simulink library "inp"  (R2021b)
settings: Solver=VariableStepAuto  StartTime=0.0  StopTime=10.0  RelTol=1e-3
undefined symbols (not defined in the file): C_TASK_5MS_S, FALSE, KINP_AcoreReadyToSlp_flg_ovrdflg, KINP_AcoreReadyToSlp_flg_ovrdval, KINP_AllowMovThd_OTA_enum_ovrdflg, KINP_AllowMovThd_OTA_enum_ovrdval, KINP_APSAngleTarget_Deg_ovrdflg, KINP_APSAngleTarget_Deg_ovrdval, KINP_APSDecReq_mps2_ovrdflg, KINP_APSDecReq_mps2_ovrdval, KINP_APSDecReqA_flg_ovrdflg, KINP_APSDecReqA_flg_ovrdval, KINP_APSDFLL_cm_ovrdflg, KINP_APSDFLL_cm_ovrdval, KINP_APSDFLR_cm_ovrdflg, KINP_APSDFLR_cm_ovrdval, KINP_APSDRLL_cm_ovrdflg, KINP_APSDRLL_cm_ovrdval, KINP_APSDRLR_cm_ovrdflg, KINP_APSDRLR_cm_ovrdval, KINP_APSExitCondition_enum_ovrdflg, KINP_APSExitCondition_enum_ovrdval, KINP_APSHWVer_enum_ovrdflg, KINP_APSHWVer_enum_ovrdval, KINP_APSProgressPCT_pct_ovrdflg, KINP_APSProgressPCT_pct_ovrdval, KINP_APSPwrReq_enum_ovrdflg, KINP_APSPwrReq_enum_ovrdval, KINP_APSReq_enum_ovrdflg, KINP_APSReq_enum_ovrdval, KINP_APSRQDisplay_enum_ovrdflg, KINP_APSRQDisplay_enum_ovrdval, KINP_APSRqEPASCtrl_flg_ovrdflg, KINP_APSRqEPASCtrl_flg_ovrdval, KINP_APSShiftPosnReq_enum_ovrdval, KINP_APSShiftPosnReq_enum_ovrflg, KINP_APSSpeedCMD_kph_ovrdval, KINP_APSSpeedCMD_kph_ovrflg, KINP_APSStaSystem_enum_ovrdflg, KINP_APSStaSystem_enum_ovrdval, KINP_APSSWVer_enum_ovrdflg, KINP_APSSWVer_enum_ovrdval, KINP_APSVMCReqA_flg_ovrdval, KINP_APSVMCReqA_flg_ovrflg, KINP_APSVRqEPASCtrl_flg_ovrdflg, KINP_APSVRqEPASCtrl_flg_ovrdval, KINP_AuxBattVolmV_mV_ovrdflg, KINP_AuxBattVolmV_mV_ovrdval, KINP_CAASSta_enum_ovrdflg, KINP_CAASSta_enum_ovrdval, KINP_CAASVMCReqA_flg_ovrdval, KINP_CAASVMCReqA_flg_ovrflg, KINP_CAN1BusOff_flg_ovrdflg, KINP_CAN1BusOff_flg_ovrdval, KINP_CAN2BusOff_flg_ovrdflg, KINP_CAN2BusOff_flg_ovrdval, KINP_CAN3BusOff_flg_ovrdflg, KINP_CAN3BusOff_flg_ovrdval, KINP_CAN4BusOff_flg_ovrdflg, KINP_CAN4BusOff_flg_ovrdval ... (+152)
libraries: FVT_lib x1037, hcu_lib x1
(part 16 of 34)

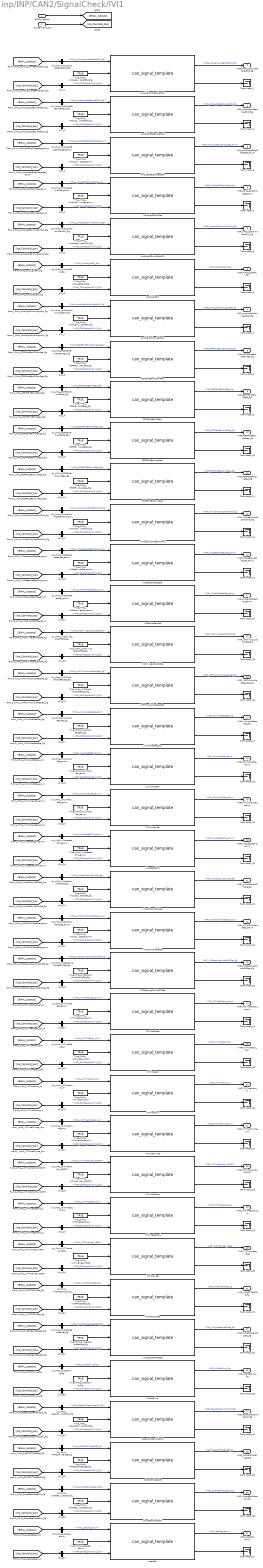
== system inp/INP/CAN2/SignalCheck/IVI1 ==
  BHAL_outputs : Inport
  inp_CanValid_bus : Inport  Port=2
  AmbLighLowBatAlertSW : FVT_lib/inp/can_signal_template  SystemSampleTime=-1  VariantActivationTime=update diagram  Latency=0  AutoFrameSizeCalculation=off
      link override defval: Value=KINP_AmbLighLowBatAlertSW_flg_defval
      link override ovrdflg: Value=KINP_AmbLighLowBatAlertSW_flg_ovrdflg
      link override ovrdval: Value=KINP_AmbLighLowBatAlertSW_flg_ovrdval
  AmbLighSafetyAlertSW : FVT_lib/inp/can_signal_template  SystemSampleTime=-1  VariantActivationTime=update diagram  Latency=0  AutoFrameSizeCalculation=off
      link override defval: Value=KINP_AmbLighSafetyAlertSW_flg_defval
      link override ovrdflg: Value=KINP_AmbLighSafetyAlertSW_flg_ovrdflg
      link override ovrdval: Value=KINP_AmbLighSafetyAlertSW_flg_ovrdval
  AmbLightBrightnessSet : FVT_lib/inp/can_signal_template  SystemSampleTime=-1  VariantActivationTime=update diagram  Latency=0  AutoFrameSizeCalculation=off
      link override defval: Value=KINP_AmbLightBrightnessSet_enum_defval
      link override ovrdflg: Value=KINP_AmbLightBrightnessSet_enum_ovrdflg
      link override ovrdval: Value=KINP_AmbLightBrightnessSet_enum_ovrdval
  AmbLightColorSet : FVT_lib/inp/can_signal_template  SystemSampleTime=-1  VariantActivationTime=update diagram  Latency=0  AutoFrameSizeCalculation=off
      link override defval: Value=KINP_AmbLightColorSet_enum_defval
      link override ovrdflg: Value=KINP_AmbLightColorSet_enum_ovrdflg
      link override ovrdval: Value=KINP_AmbLightColorSet_enum_ovrdval
  AmbLightDimInDarkSW : FVT_lib/inp/can_signal_template  SystemSampleTime=-1  VariantActivationTime=update diagram  Latency=0  AutoFrameSizeCalculation=off
      link override defval: Value=KINP_AmbLightDimInDarkSW_flg_defval
      link override ovrdflg: Value=KINP_AmbLightDimInDarkSW_flg_ovrdflg
      link override ovrdval: Value=KINP_AmbLightDimInDarkSW_flg_ovrdval
  AmbLightSW : FVT_lib/inp/can_signal_template  SystemSampleTime=-1  VariantActivationTime=update diagram  Latency=0  AutoFrameSizeCalculation=off
      link override defval: Value=KINP_AmbLightSW_flg_defval
      link override ovrdflg: Value=KINP_AmbLightSW_flg_ovrdflg
      link override ovrdval: Value=KINP_AmbLightSW_flg_ovrdval
  AmbLightWlcmLightSW : FVT_lib/inp/can_signal_template  SystemSampleTime=-1  VariantActivationTime=update diagram  Latency=0  AutoFrameSizeCalculation=off
      link override defval: Value=KINP_AmbLightWlcmLightSW_flg_defval
      link override ovrdflg: Value=KINP_AmbLightWlcmLightSW_flg_ovrdflg
      link override ovrdval: Value=KINP_AmbLightWlcmLightSW_flg_ovrdval
  FCPFrEvtBtnACMaxReq : FVT_lib/inp/can_signal_template  SystemSampleTime=-1  VariantActivationTime=update diagram  Latency=0  AutoFrameSizeCalculation=off
      link override defval: Value=KINP_FCPFrEvtBtnACMaxReq_flg_defval
      link override ovrdflg: Value=KINP_FCPFrEvtBtnACMaxReq_flg_ovrdflg
      link override ovrdval: Value=KINP_FCPFrEvtBtnACMaxReq_flg_ovrdval
  FCPFrEvtBtnACReq : FVT_lib/inp/can_signal_template  SystemSampleTime=-1  VariantActivationTime=update diagram  Latency=0  AutoFrameSizeCalculation=off
      link override defval: Value=KINP_FCPFrEvtBtnACReq_flg_defval
      link override ovrdflg: Value=KINP_FCPFrEvtBtnACReq_flg_ovrdflg
      link override ovrdval: Value=KINP_FCPFrEvtBtnACReq_flg_ovrdval
  FCPFrEvtBtnAutoReq : FVT_lib/inp/can_signal_template  SystemSampleTime=-1  VariantActivationTime=update diagram  Latency=0  AutoFrameSizeCalculation=off
      link override defval: Value=KINP_FCPFrEvtBtnAutoReq_flg_defval
      link override ovrdflg: Value=KINP_FCPFrEvtBtnAutoReq_flg_ovrdflg
      link override ovrdval: Value=KINP_FCPFrEvtBtnAutoReq_flg_ovrdval
  FCPFrEvtBtnSyncReq : FVT_lib/inp/can_signal_template  SystemSampleTime=-1  VariantActivationTime=update diagram  Latency=0  AutoFrameSizeCalculation=off
      link override defval: Value=KINP_FCPFrEvtBtnSyncReq_flg_defval
      link override ovrdflg: Value=KINP_FCPFrEvtBtnSyncReq_flg_ovrdflg
      link override ovrdval: Value=KINP_FCPFrEvtBtnSyncReq_flg_ovrdval
  IVIAutoWipHSpdSWCmd : FVT_lib/inp/can_signal_template  SystemSampleTime=-1  VariantActivationTime=update diagram  Latency=0  AutoFrameSizeCalculation=off
      link override defval: Value=KINP_IVIAutoWipHSpdSWCmd_flg_defval
      link override ovrdflg: Value=KINP_IVIAutoWipHSpdSWCmd_flg_ovrdflg
      link override ovrdval: Value=KINP_IVIAutoWipHSpdSWCmd_flg_ovrdval
  IVICreateAccReqSta : FVT_lib/inp/can_signal_template  SystemSampleTime=-1  VariantActivationTime=update diagram  Latency=0  AutoFrameSizeCalculation=off
      link override defval: Value=KINP_IVICreateAccReqSta_enum_defval
      link override ovrdflg: Value=KINP_IVICreateAccReqSta_enum_ovrdflg
      link override ovrdval: Value=KINP_IVICreateAccReqSta_enum_ovrdval
  IVIDelAccReqSta : FVT_lib/inp/can_signal_template  SystemSampleTime=-1  VariantActivationTime=update diagram  Latency=0  AutoFrameSizeCalculation=off
      link override defval: Value=KINP_IVIDelAccReqSta_enum_defval
      link override ovrdflg: Value=KINP_IVIDelAccReqSta_enum_ovrdflg
      link override ovrdval: Value=KINP_IVIDelAccReqSta_enum_ovrdval
  IVIDrivingLockSWSta : FVT_lib/inp/can_signal_template  SystemSampleTime=-1  VariantActivationTime=update diagram  Latency=0  AutoFrameSizeCalculation=off
      link override defval: Value=KINP_IVIDrivingLockSWSta_flg_defval
      link override ovrdflg: Value=KINP_IVIDrivingLockSWSta_flg_ovrdflg
      link override ovrdval: Value=KINP_IVIDrivingLockSWSta_flg_ovrdval
  IVIFrTrunkUnlockReqSta : FVT_lib/inp/can_signal_template  SystemSampleTime=-1  VariantActivationTime=update diagram  Latency=0  AutoFrameSizeCalculation=off
      link override defval: Value=KINP_IVIFrTrunkUnlockReqSta_flg_defval
      link override ovrdflg: Value=KINP_IVIFrTrunkUnlockReqSta_flg_ovrdflg
      link override ovrdval: Value=KINP_IVIFrTrunkUnlockReqSta_flg_ovrdval
  IVILinkAccReqSta : FVT_lib/inp/can_signal_template  SystemSampleTime=-1  VariantActivationTime=update diagram  Latency=0  AutoFrameSizeCalculation=off
      link override defval: Value=KINP_IVILinkAccReqSta_flg_defval
      link override ovrdflg: Value=KINP_IVILinkAccReqSta_flg_ovrdflg
      link override ovrdval: Value=KINP_IVILinkAccReqSta_flg_ovrdval
  IVILinkAccSta : FVT_lib/inp/can_signal_template  SystemSampleTime=-1  VariantActivationTime=update diagram  Latency=0  AutoFrameSizeCalculation=off
      link override defval: Value=KINP_IVILinkAccSta_enum_defval
      link override ovrdflg: Value=KINP_IVILinkAccSta_enum_ovrdflg
      link override ovrdval: Value=KINP_IVILinkAccSta_enum_ovrdval
  IVILinkKeySta : FVT_lib/inp/can_signal_template  SystemSampleTime=-1  VariantActivationTime=update diagram  Latency=0  AutoFrameSizeCalculation=off
      link override defval: Value=KINP_IVILinkKeySta_enum_defval
      link override ovrdflg: Value=KINP_IVILinkKeySta_enum_ovrdflg
      link override ovrdval: Value=KINP_IVILinkKeySta_enum_ovrdval
  IVILocatedSTA : FVT_lib/inp/can_signal_template  SystemSampleTime=-1  VariantActivationTime=update diagram  Latency=0  AutoFrameSizeCalculation=off
      link override defval: Value=KINP_IVILocatedSTA_enum_defval
      link override ovrdflg: Value=KINP_IVILocatedSTA_enum_ovrdflg
      link override ovrdval: Value=KINP_IVILocatedSTA_enum_ovrdval
  IVILockSoundSWSta : FVT_lib/inp/can_signal_template  SystemSampleTime=-1  VariantActivationTime=update diagram  Latency=0  AutoFrameSizeCalculation=off
      link override defval: Value=KINP_IVILockSoundSWSta_flg_defval
      link override ovrdflg: Value=KINP_IVILockSoundSWSta_flg_ovrdflg
      link override ovrdval: Value=KINP_IVILockSoundSWSta_flg_ovrdval
  IVISWCVibModeSta : FVT_lib/inp/can_signal_template  SystemSampleTime=-1  VariantActivationTime=update diagram  Latency=0  AutoFrameSizeCalculation=off
      link override defval: Value=KINP_IVISWCVibModeSta_enum_defval
      link override ovrdflg: Value=KINP_IVISWCVibModeSta_enum_ovrdflg
      link override ovrdval: Value=KINP_IVISWCVibModeSta_enum_ovrdval
  IVIStoppingUnlockSWSta : FVT_lib/inp/can_signal_template  SystemSampleTime=-1  VariantActivationTime=update diagram  Latency=0  AutoFrameSizeCalculation=off
      link override defval: Value=KINP_IVIStoppingUnlockSWSta_flg_defval
      link override ovrdflg: Value=KINP_IVIStoppingUnlockSWSta_flg_ovrdflg
      link override ovrdval: Value=KINP_IVIStoppingUnlockSWSta_flg_ovrdval
  IVITimeCheck : FVT_lib/inp/can_signal_template  SystemSampleTime=-1  VariantActivationTime=update diagram  Latency=0  AutoFrameSizeCalculation=off
      link override defval: Value=KINP_IVITimeCheck_enum_defval
      link override ovrdflg: Value=KINP_IVITimeCheck_enum_ovrdflg
      link override ovrdval: Value=KINP_IVITimeCheck_enum_ovrdval
  IVITimeDay : FVT_lib/inp/can_signal_template  SystemSampleTime=-1  VariantActivationTime=update diagram  Latency=0  AutoFrameSizeCalculation=off
      link override defval: Value=KINP_IVITimeDay_DAY_defval
      link override ovrdflg: Value=KINP_IVITimeDay_DAY_ovrdflg
      link override ovrdval: Value=KINP_IVITimeDay_DAY_ovrdval
  IVITimeHour : FVT_lib/inp/can_signal_template  SystemSampleTime=-1  VariantActivationTime=update diagram  Latency=0  AutoFrameSizeCalculation=off
      link override defval: Value=KINP_IVITimeHour_hr_defval
      link override ovrdflg: Value=KINP_IVITimeHour_hr_ovrdflg
      link override ovrdval: Value=KINP_IVITimeHour_hr_ovrdval
  IVITimeMinute : FVT_lib/inp/can_signal_template  SystemSampleTime=-1  VariantActivationTime=update diagram  Latency=0  AutoFrameSizeCalculation=off
      link override defval: Value=KINP_IVITimeMinute_min_defval
      link override ovrdflg: Value=KINP_IVITimeMinute_min_ovrdflg
      link override ovrdval: Value=KINP_IVITimeMinute_min_ovrdval
  IVITimeMonth : FVT_lib/inp/can_signal_template  SystemSampleTime=-1  VariantActivationTime=update diagram  Latency=0  AutoFrameSizeCalculation=off
      link override defval: Value=KINP_IVITimeMonth_MONTH_defval
      link override ovrdflg: Value=KINP_IVITimeMonth_MONTH_ovrdflg
      link override ovrdval: Value=KINP_IVITimeMonth_MONTH_ovrdval
  IVITimeSecond : FVT_lib/inp/can_signal_template  SystemSampleTime=-1  VariantActivationTime=update diagram  Latency=0  AutoFrameSizeCalculation=off
      link override defval: Value=KINP_IVITimeSecond_s_defval
      link override ovrdflg: Value=KINP_IVITimeSecond_s_ovrdflg
      link override ovrdval: Value=KINP_IVITimeSecond_s_ovrdval
  IVITimeYear : FVT_lib/inp/can_signal_template  SystemSampleTime=-1  VariantActivationTime=update diagram  Latency=0  AutoFrameSizeCalculation=off
      link override defval: Value=KINP_IVITimeYear_YEAR_defval
      link override ovrdflg: Value=KINP_IVITimeYear_YEAR_ovrdflg
      link override ovrdval: Value=KINP_IVITimeYear_YEAR_ovrdval
  IVIWPTCSWSta : FVT_lib/inp/can_signal_template  SystemSampleTime=-1  VariantActivationTime=update diagram  Latency=0  AutoFrameSizeCalculation=off
      link override defval: Value=KINP_IVIWPTCSWSta_flg_defval
      link override ovrdflg: Value=KINP_IVIWPTCSWSta_flg_ovrdflg
      link override ovrdval: Value=KINP_IVIWPTCSWSta_flg_ovrdval
  IVIsigScreenReqSta : FVT_lib/inp/can_signal_template  SystemSampleTime=-1  VariantActivationTime=update diagram  Latency=0  AutoFrameSizeCalculation=off
      link override defval: Value=KINP_IVIsigScreenReqSta_flg_defval
      link override ovrdflg: Value=KINP_IVIsigScreenReqSta_flg_ovrdflg
      link override ovrdval: Value=KINP_IVIsigScreenReqSta_flg_ovrdval
  LINKtoDrive : FVT_lib/inp/can_signal_template  SystemSampleTime=-1  VariantActivationTime=update diagram  Latency=0  AutoFrameSizeCalculation=off
      link override defval: Value=KINP_LINKtoDrive_flg_defval
      link override ovrdflg: Value=KINP_LINKtoDrive_flg_ovrdflg
      link override ovrdval: Value=KINP_LINKtoDrive_flg_ovrdval
  OpenDrOpenWdoSW : FVT_lib/inp/can_signal_template  SystemSampleTime=-1  VariantActivationTime=update diagram  Latency=0  AutoFrameSizeCalculation=off
      link override defval: Value=KINP_OpenDrOpenWdoSW_flg_defval
      link override ovrdflg: Value=KINP_OpenDrOpenWdoSW_flg_ovrdflg
      link override ovrdval: Value=KINP_OpenDrOpenWdoSW_flg_ovrdval
  PWCONTINUEUSE : FVT_lib/inp/can_signal_template  SystemSampleTime=-1  VariantActivationTime=update diagram  Latency=0  AutoFrameSizeCalculation=off
      link override defval: Value=KINP_PWCONTINUEUSE_flg_defval
      link override ovrdflg: Value=KINP_PWCONTINUEUSE_flg_ovrdflg
      link override ovrdval: Value=KINP_PWCONTINUEUSE_flg_ovrdval
  SmartEcoModeSW : FVT_lib/inp/can_signal_template  SystemSampleTime=-1  VariantActivationTime=update diagram  Latency=0  AutoFrameSizeCalculation=off
      link override defval: Value=KINP_SmartEcoModeSW_flg_defval
      link override ovrdflg: Value=KINP_SmartEcoModeSW_flg_ovrdflg
      link override ovrdval: Value=KINP_SmartEcoModeSW_flg_ovrdval
  Terminator_{1..37} (37 alike) : Terminator
  True_VHAL_AmbLighLowBatAlertSW_flg : Constant  Value=TRUE  OutDataTypeStr=boolean
  True_VHAL_AmbLighSafetyAlertSW_flg : Constant  Value=TRUE  OutDataTypeStr=boolean
  True_VHAL_AmbLightBrightnessSet_enum : Constant  Value=TRUE  OutDataTypeStr=boolean
  True_VHAL_AmbLightColorSet_enum : Constant  Value=TRUE  OutDataTypeStr=boolean
  True_VHAL_AmbLightDimInDarkSW_flg : Constant  Value=TRUE  OutDataTypeStr=boolean
  True_VHAL_AmbLightSW_flg : Constant  Value=TRUE  OutDataTypeStr=boolean
  True_VHAL_AmbLightWlcmLightSW_flg : Constant  Value=TRUE  OutDataTypeStr=boolean
  True_VHAL_FCPFrEvtBtnACMaxReq_flg : Constant  Value=TRUE  OutDataTypeStr=boolean
  True_VHAL_FCPFrEvtBtnACReq_flg : Constant  Value=TRUE  OutDataTypeStr=boolean
  True_VHAL_FCPFrEvtBtnAutoReq_flg : Constant  Value=TRUE  OutDataTypeStr=boolean
  True_VHAL_FCPFrEvtBtnSyncReq_flg : Constant  Value=TRUE  OutDataTypeStr=boolean
  True_VHAL_IVIAutoWipHSpdSWCmd_flg : Constant  Value=TRUE  OutDataTypeStr=boolean
  True_VHAL_IVICreateAccReqSta_enum : Constant  Value=TRUE  OutDataTypeStr=boolean
  True_VHAL_IVIDelAccReqSta_enum : Constant  Value=TRUE  OutDataTypeStr=boolean
  True_VHAL_IVIDrivingLockSWSta_flg : Constant  Value=TRUE  OutDataTypeStr=boolean
  True_VHAL_IVIFrTrunkUnlockReqSta_flg : Constant  Value=TRUE  OutDataTypeStr=boolean
  True_VHAL_IVILinkAccReqSta_flg : Constant  Value=TRUE  OutDataTypeStr=boolean
  True_VHAL_IVILinkAccSta_enum : Constant  Value=TRUE  OutDataTypeStr=boolean
  True_VHAL_IVILinkKeySta_enum : Constant  Value=TRUE  OutDataTypeStr=boolean
  True_VHAL_IVILocatedSTA_enum : Constant  Value=TRUE  OutDataTypeStr=boolean
  True_VHAL_IVILockSoundSWSta_flg : Constant  Value=TRUE  OutDataTypeStr=boolean
  True_VHAL_IVISWCVibModeSta_enum : Constant  Value=TRUE  OutDataTypeStr=boolean
  True_VHAL_IVIStoppingUnlockSWSta_flg : Constant  Value=TRUE  OutDataTypeStr=boolean
  True_VHAL_IVITimeCheck_enum : Constant  Value=TRUE  OutDataTypeStr=boolean
  True_VHAL_IVITimeDay_DAY : Constant  Value=TRUE  OutDataTypeStr=boolean
  True_VHAL_IVITimeHour_hr : Constant  Value=TRUE  OutDataTypeStr=boolean
  True_VHAL_IVITimeMinute_min : Constant  Value=TRUE  OutDataTypeStr=boolean
  True_VHAL_IVITimeMonth_MONTH : Constant  Value=TRUE  OutDataTypeStr=boolean
  True_VHAL_IVITimeSecond_s : Constant  Value=TRUE  OutDataTypeStr=boolean
  True_VHAL_IVITimeYear_YEAR : Constant  Value=TRUE  OutDataTypeStr=boolean
  True_VHAL_IVIWPTCSWSta_flg : Constant  Value=TRUE  OutDataTypeStr=boolean
  True_VHAL_IVIsigScreenReqSta_flg : Constant  Value=TRUE  OutDataTypeStr=boolean
  True_VHAL_LINKtoDrive_flg : Constant  Value=TRUE  OutDataTypeStr=boolean
  True_VHAL_OpenDrOpenWdoSW_flg : Constant  Value=TRUE  OutDataTypeStr=boolean
  True_VHAL_PWCONTINUEUSE_flg : Constant  Value=TRUE  OutDataTypeStr=boolean
  True_VHAL_SmartEcoModeSW_flg : Constant  Value=TRUE  OutDataTypeStr=boolean
  True_VHAL_UserSet_enum : Constant  Value=TRUE  OutDataTypeStr=boolean
  UserSet : FVT_lib/inp/can_signal_template  SystemSampleTime=-1  VariantActivationTime=update diagram  Latency=0  AutoFrameSizeCalculation=off
      link override defval: Value=KINP_UserSet_enum_defval
      link override ovrdflg: Value=KINP_UserSet_enum_ovrdflg
      link override ovrdval: Value=KINP_UserSet_enum_ovrdval
  slr1_{1..37} (37 alike) : BusSelector  OutputSignals=VINP_CANMsgValidIVI1_flg
  slr_VHAL_AmbLighLowBatAlertSW_flg : BusSelector  OutputSignals=VHAL_AmbLighLowBatAlertSW_flg
  slr_VHAL_AmbLighSafetyAlertSW_flg : BusSelector  OutputSignals=VHAL_AmbLighSafetyAlertSW_flg
  slr_VHAL_AmbLightBrightnessSet_enum : BusSelector  OutputSignals=VHAL_AmbLightBrightnessSet_enum
  slr_VHAL_AmbLightColorSet_enum : BusSelector  OutputSignals=VHAL_AmbLightColorSet_enum
  slr_VHAL_AmbLightDimInDarkSW_flg : BusSelector  OutputSignals=VHAL_AmbLightDimInDarkSW_flg
  slr_VHAL_AmbLightSW_flg : BusSelector  OutputSignals=VHAL_AmbLightSW_flg
  slr_VHAL_AmbLightWlcmLightSW_flg : BusSelector  OutputSignals=VHAL_AmbLightWlcmLightSW_flg
  slr_VHAL_FCPFrEvtBtnACMaxReq_flg : BusSelector  OutputSignals=VHAL_FCPFrEvtBtnACMaxReq_flg
  slr_VHAL_FCPFrEvtBtnACReq_flg : BusSelector  OutputSignals=VHAL_FCPFrEvtBtnACReq_flg
  slr_VHAL_FCPFrEvtBtnAutoReq_flg : BusSelector  OutputSignals=VHAL_FCPFrEvtBtnAutoReq_flg
  slr_VHAL_FCPFrEvtBtnSyncReq_flg : BusSelector  OutputSignals=VHAL_FCPFrEvtBtnSyncReq_flg
  slr_VHAL_IVIAutoWipHSpdSWCmd_flg : BusSelector  OutputSignals=VHAL_IVIAutoWipHSpdSWCmd_flg
  slr_VHAL_IVICreateAccReqSta_enum : BusSelector  OutputSignals=VHAL_IVICreateAccReqSta_enum
  slr_VHAL_IVIDelAccReqSta_enum : BusSelector  OutputSignals=VHAL_IVIDelAccReqSta_enum
  slr_VHAL_IVIDrivingLockSWSta_flg : BusSelector  OutputSignals=VHAL_IVIDrivingLockSWSta_flg
  slr_VHAL_IVIFrTrunkUnlockReqSta_flg : BusSelector  OutputSignals=VHAL_IVIFrTrunkUnlockReqSta_flg
  slr_VHAL_IVILinkAccReqSta_flg : BusSelector  OutputSignals=VHAL_IVILinkAccReqSta_flg
  slr_VHAL_IVILinkAccSta_enum : BusSelector  OutputSignals=VHAL_IVILinkAccSta_enum
  slr_VHAL_IVILinkKeySta_enum : BusSelector  OutputSignals=VHAL_IVILinkKeySta_enum
  slr_VHAL_IVILocatedSTA_enum : BusSelector  OutputSignals=VHAL_IVILocatedSTA_enum
  slr_VHAL_IVILockSoundSWSta_flg : BusSelector  OutputSignals=VHAL_IVILockSoundSWSta_flg
  slr_VHAL_IVISWCVibModeSta_enum : BusSelector  OutputSignals=VHAL_IVISWCVibModeSta_enum
  slr_VHAL_IVIStoppingUnlockSWSta_flg : BusSelector  OutputSignals=VHAL_IVIStoppingUnlockSWSta_flg
  slr_VHAL_IVITimeCheck_enum : BusSelector  OutputSignals=VHAL_IVITimeCheck_enum
  slr_VHAL_IVITimeDay_DAY : BusSelector  OutputSignals=VHAL_IVITimeDay_DAY
  slr_VHAL_IVITimeHour_hr : BusSelector  OutputSignals=VHAL_IVITimeHour_hr
  slr_VHAL_IVITimeMinute_min : BusSelector  OutputSignals=VHAL_IVITimeMinute_min
  slr_VHAL_IVITimeMonth_MONTH : BusSelector  OutputSignals=VHAL_IVITimeMonth_MONTH
  slr_VHAL_IVITimeSecond_s : BusSelector  OutputSignals=VHAL_IVITimeSecond_s
  slr_VHAL_IVITimeYear_YEAR : BusSelector  OutputSignals=VHAL_IVITimeYear_YEAR
  slr_VHAL_IVIWPTCSWSta_flg : BusSelector  OutputSignals=VHAL_IVIWPTCSWSta_flg
  slr_VHAL_IVIsigScreenReqSta_flg : BusSelector  OutputSignals=VHAL_IVIsigScreenReqSta_flg
  slr_VHAL_LINKtoDrive_flg : BusSelector  OutputSignals=VHAL_LINKtoDrive_flg
  slr_VHAL_OpenDrOpenWdoSW_flg : BusSelector  OutputSignals=VHAL_OpenDrOpenWdoSW_flg
  slr_VHAL_PWCONTINUEUSE_flg : BusSelector  OutputSignals=VHAL_PWCONTINUEUSE_flg
  slr_VHAL_SmartEcoModeSW_flg : BusSelector  OutputSignals=VHAL_SmartEcoModeSW_flg
  slr_VHAL_UserSet_enum : BusSelector  OutputSignals=VHAL_UserSet_enum
  VINP_AmbLighLowBatAlertSW_flg : Outport
  VINP_AmbLighSafetyAlertSW_flg : Outport  Port=2
  VINP_AmbLightBrightnessSet_enum : Outport  Port=3
  VINP_AmbLightColorSet_enum : Outport  Port=4
  VINP_AmbLightDimInDarkSW_flg : Outport  Port=5
  VINP_AmbLightSW_flg : Outport  Port=6
  VINP_AmbLightWlcmLightSW_flg : Outport  Port=7
  VINP_FCPFrEvtBtnACMaxReq_flg : Outport  Port=8
  VINP_FCPFrEvtBtnACReq_flg : Outport  Port=9
  VINP_FCPFrEvtBtnAutoReq_flg : Outport  Port=10
  VINP_FCPFrEvtBtnSyncReq_flg : Outport  Port=11
  VINP_IVIAutoWipHSpdSWCmd_flg : Outport  Port=12
  VINP_IVICreateAccReqSta_enum : Outport  Port=13
  VINP_IVIDelAccReqSta_enum : Outport  Port=14
  VINP_IVIDrivingLockSWSta_flg : Outport  Port=15
  VINP_IVIFrTrunkUnlockReqSta_flg : Outport  Port=16
  VINP_IVILinkAccReqSta_flg : Outport  Port=17
  VINP_IVILinkAccSta_enum : Outport  Port=18
  VINP_IVILinkKeySta_enum : Outport  Port=19
  VINP_IVILocatedSTA_enum : Outport  Port=20
  VINP_IVILockSoundSWSta_flg : Outport  Port=21
  VINP_IVISWCVibModeSta_enum : Outport  Port=22
  VINP_IVIStoppingUnlockSWSta_flg : Outport  Port=23
  VINP_IVITimeCheck_enum : Outport  Port=24
  VINP_IVITimeDay_DAY : Outport  Port=25
  VINP_IVITimeHour_hr : Outport  Port=26
  VINP_IVITimeMinute_min : Outport  Port=27
  VINP_IVITimeMonth_MONTH : Outport  Port=28
  VINP_IVITimeSecond_s : Outport  Port=29
  VINP_IVITimeYear_YEAR : Outport  Port=30
  VINP_IVIWPTCSWSta_flg : Outport  Port=31
  VINP_IVIsigScreenReqSta_flg : Outport  Port=32
  VINP_LINKtoDrive_flg : Outport  Port=33
  VINP_OpenDrOpenWdoSW_flg : Outport  Port=34
  VINP_PWCONTINUEUSE_flg : Outport  Port=35
  VINP_SmartEcoModeSW_flg : Outport  Port=36
  VINP_UserSet_enum : Outport  Port=37
  wires:
  BHAL_outputs/1 -> [BHAL_outputs]
  inp_CanValid_bus/1 -> [inp_CanValid_bus]
  [BHAL_outputs] -> slr_VHAL_AmbLighLowBatAlertSW_flg/1
  slr_VHAL_AmbLighLowBatAlertSW_flg/1 -> AmbLighLowBatAlertSW/1  "<VHAL_AmbLighLowBatAlertSW_flg>"
  True_VHAL_AmbLighLowBatAlertSW_flg/1 -> AmbLighLowBatAlertSW/2
  [inp_CanValid_bus] -> slr1_1/1
  slr1_1/1 -> AmbLighLowBatAlertSW/3  "<VINP_CANMsgValidIVI1_flg>"
  AmbLighLowBatAlertSW/1 -> VINP_AmbLighLowBatAlertSW_flg/1  "VINP_AmbLighLowBatAlertSW_flg"
  AmbLighLowBatAlertSW/2 -> Terminator_1/1
  [BHAL_outputs] -> slr_VHAL_AmbLighSafetyAlertSW_flg/1
  slr_VHAL_AmbLighSafetyAlertSW_flg/1 -> AmbLighSafetyAlertSW/1  "<VHAL_AmbLighSafetyAlertSW_flg>"
  True_VHAL_AmbLighSafetyAlertSW_flg/1 -> AmbLighSafetyAlertSW/2
  [inp_CanValid_bus] -> slr1_2/1
  slr1_2/1 -> AmbLighSafetyAlertSW/3  "<VINP_CANMsgValidIVI1_flg>"
  AmbLighSafetyAlertSW/1 -> VINP_AmbLighSafetyAlertSW_flg/1  "VINP_AmbLighSafetyAlertSW_flg"
  AmbLighSafetyAlertSW/2 -> Terminator_2/1
  [BHAL_outputs] -> slr_VHAL_AmbLightBrightnessSet_enum/1
  slr_VHAL_AmbLightBrightnessSet_enum/1 -> AmbLightBrightnessSet/1  "<VHAL_AmbLightBrightnessSet_enum>"
  True_VHAL_AmbLightBrightnessSet_enum/1 -> AmbLightBrightnessSet/2
  [inp_CanValid_bus] -> slr1_3/1
  slr1_3/1 -> AmbLightBrightnessSet/3  "<VINP_CANMsgValidIVI1_flg>"
  AmbLightBrightnessSet/1 -> VINP_AmbLightBrightnessSet_enum/1  "VINP_AmbLightBrightnessSet_enum"
  AmbLightBrightnessSet/2 -> Terminator_3/1
  [BHAL_outputs] -> slr_VHAL_AmbLightColorSet_enum/1
  slr_VHAL_AmbLightColorSet_enum/1 -> AmbLightColorSet/1  "<VHAL_AmbLightColorSet_enum>"
  True_VHAL_AmbLightColorSet_enum/1 -> AmbLightColorSet/2
  [inp_CanValid_bus] -> slr1_4/1
  slr1_4/1 -> AmbLightColorSet/3  "<VINP_CANMsgValidIVI1_flg>"
  AmbLightColorSet/1 -> VINP_AmbLightColorSet_enum/1  "VINP_AmbLightColorSet_enum"
  AmbLightColorSet/2 -> Terminator_4/1
  [BHAL_outputs] -> slr_VHAL_AmbLightDimInDarkSW_flg/1
  slr_VHAL_AmbLightDimInDarkSW_flg/1 -> AmbLightDimInDarkSW/1  "<VHAL_AmbLightDimInDarkSW_flg>"
  True_VHAL_AmbLightDimInDarkSW_flg/1 -> AmbLightDimInDarkSW/2
  [inp_CanValid_bus] -> slr1_5/1
  slr1_5/1 -> AmbLightDimInDarkSW/3  "<VINP_CANMsgValidIVI1_flg>"
  AmbLightDimInDarkSW/1 -> VINP_AmbLightDimInDarkSW_flg/1  "VINP_AmbLightDimInDarkSW_flg"
  AmbLightDimInDarkSW/2 -> Terminator_5/1
  [BHAL_outputs] -> slr_VHAL_AmbLightSW_flg/1
  slr_VHAL_AmbLightSW_flg/1 -> AmbLightSW/1  "<VHAL_AmbLightSW_flg>"
  True_VHAL_AmbLightSW_flg/1 -> AmbLightSW/2
  [inp_CanValid_bus] -> slr1_6/1
  slr1_6/1 -> AmbLightSW/3  "<VINP_CANMsgValidIVI1_flg>"
  AmbLightSW/1 -> VINP_AmbLightSW_flg/1  "VINP_AmbLightSW_flg"
  AmbLightSW/2 -> Terminator_6/1
  [BHAL_outputs] -> slr_VHAL_AmbLightWlcmLightSW_flg/1
  slr_VHAL_AmbLightWlcmLightSW_flg/1 -> AmbLightWlcmLightSW/1  "<VHAL_AmbLightWlcmLightSW_flg>"
  True_VHAL_AmbLightWlcmLightSW_flg/1 -> AmbLightWlcmLightSW/2
  [inp_CanValid_bus] -> slr1_7/1
  slr1_7/1 -> AmbLightWlcmLightSW/3  "<VINP_CANMsgValidIVI1_flg>"
  AmbLightWlcmLightSW/1 -> VINP_AmbLightWlcmLightSW_flg/1  "VINP_AmbLightWlcmLightSW_flg"
  AmbLightWlcmLightSW/2 -> Terminator_7/1
  [BHAL_outputs] -> slr_VHAL_FCPFrEvtBtnACMaxReq_flg/1
  slr_VHAL_FCPFrEvtBtnACMaxReq_flg/1 -> FCPFrEvtBtnACMaxReq/1  "<VHAL_FCPFrEvtBtnACMaxReq_flg>"
  True_VHAL_FCPFrEvtBtnACMaxReq_flg/1 -> FCPFrEvtBtnACMaxReq/2
  [inp_CanValid_bus] -> slr1_8/1
  slr1_8/1 -> FCPFrEvtBtnACMaxReq/3  "<VINP_CANMsgValidIVI1_flg>"
  FCPFrEvtBtnACMaxReq/1 -> VINP_FCPFrEvtBtnACMaxReq_flg/1  "VINP_FCPFrEvtBtnACMaxReq_flg"
  FCPFrEvtBtnACMaxReq/2 -> Terminator_8/1
  [BHAL_outputs] -> slr_VHAL_FCPFrEvtBtnACReq_flg/1
  slr_VHAL_FCPFrEvtBtnACReq_flg/1 -> FCPFrEvtBtnACReq/1  "<VHAL_FCPFrEvtBtnACReq_flg>"
  True_VHAL_FCPFrEvtBtnACReq_flg/1 -> FCPFrEvtBtnACReq/2
  [inp_CanValid_bus] -> slr1_9/1
  slr1_9/1 -> FCPFrEvtBtnACReq/3  "<VINP_CANMsgValidIVI1_flg>"
  FCPFrEvtBtnACReq/1 -> VINP_FCPFrEvtBtnACReq_flg/1  "VINP_FCPFrEvtBtnACReq_flg"
  FCPFrEvtBtnACReq/2 -> Terminator_9/1
  [BHAL_outputs] -> slr_VHAL_FCPFrEvtBtnAutoReq_flg/1
  slr_VHAL_FCPFrEvtBtnAutoReq_flg/1 -> FCPFrEvtBtnAutoReq/1  "<VHAL_FCPFrEvtBtnAutoReq_flg>"
  True_VHAL_FCPFrEvtBtnAutoReq_flg/1 -> FCPFrEvtBtnAutoReq/2
  [inp_CanValid_bus] -> slr1_10/1
  slr1_10/1 -> FCPFrEvtBtnAutoReq/3  "<VINP_CANMsgValidIVI1_flg>"
  FCPFrEvtBtnAutoReq/1 -> VINP_FCPFrEvtBtnAutoReq_flg/1  "VINP_FCPFrEvtBtnAutoReq_flg"
  FCPFrEvtBtnAutoReq/2 -> Terminator_10/1
  [BHAL_outputs] -> slr_VHAL_FCPFrEvtBtnSyncReq_flg/1
  slr_VHAL_FCPFrEvtBtnSyncReq_flg/1 -> FCPFrEvtBtnSyncReq/1  "<VHAL_FCPFrEvtBtnSyncReq_flg>"
  True_VHAL_FCPFrEvtBtnSyncReq_flg/1 -> FCPFrEvtBtnSyncReq/2
  [inp_CanValid_bus] -> slr1_11/1
  slr1_11/1 -> FCPFrEvtBtnSyncReq/3  "<VINP_CANMsgValidIVI1_flg>"
  FCPFrEvtBtnSyncReq/1 -> VINP_FCPFrEvtBtnSyncReq_flg/1  "VINP_FCPFrEvtBtnSyncReq_flg"
  FCPFrEvtBtnSyncReq/2 -> Terminator_11/1
  [BHAL_outputs] -> slr_VHAL_IVIAutoWipHSpdSWCmd_flg/1
  slr_VHAL_IVIAutoWipHSpdSWCmd_flg/1 -> IVIAutoWipHSpdSWCmd/1  "<VHAL_IVIAutoWipHSpdSWCmd_flg>"
  True_VHAL_IVIAutoWipHSpdSWCmd_flg/1 -> IVIAutoWipHSpdSWCmd/2
  [inp_CanValid_bus] -> slr1_12/1
  slr1_12/1 -> IVIAutoWipHSpdSWCmd/3  "<VINP_CANMsgValidIVI1_flg>"
  IVIAutoWipHSpdSWCmd/1 -> VINP_IVIAutoWipHSpdSWCmd_flg/1  "VINP_IVIAutoWipHSpdSWCmd_flg"
  IVIAutoWipHSpdSWCmd/2 -> Terminator_12/1
  [BHAL_outputs] -> slr_VHAL_IVICreateAccReqSta_enum/1
  slr_VHAL_IVICreateAccReqSta_enum/1 -> IVICreateAccReqSta/1  "<VHAL_IVICreateAccReqSta_enum>"
  True_VHAL_IVICreateAccReqSta_enum/1 -> IVICreateAccReqSta/2
  [inp_CanValid_bus] -> slr1_13/1
  slr1_13/1 -> IVICreateAccReqSta/3  "<VINP_CANMsgValidIVI1_flg>"
  IVICreateAccReqSta/1 -> VINP_IVICreateAccReqSta_enum/1  "VINP_IVICreateAccReqSta_enum"
  IVICreateAccReqSta/2 -> Terminator_13/1
  [BHAL_outputs] -> slr_VHAL_IVIDelAccReqSta_enum/1
  slr_VHAL_IVIDelAccReqSta_enum/1 -> IVIDelAccReqSta/1  "<VHAL_IVIDelAccReqSta_enum>"
  True_VHAL_IVIDelAccReqSta_enum/1 -> IVIDelAccReqSta/2
  [inp_CanValid_bus] -> slr1_14/1
  slr1_14/1 -> IVIDelAccReqSta/3  "<VINP_CANMsgValidIVI1_flg>"
  IVIDelAccReqSta/1 -> VINP_IVIDelAccReqSta_enum/1  "VINP_IVIDelAccReqSta_enum"
  IVIDelAccReqSta/2 -> Terminator_14/1
  [BHAL_outputs] -> slr_VHAL_IVIDrivingLockSWSta_flg/1
  slr_VHAL_IVIDrivingLockSWSta_flg/1 -> IVIDrivingLockSWSta/1  "<VHAL_IVIDrivingLockSWSta_flg>"
  True_VHAL_IVIDrivingLockSWSta_flg/1 -> IVIDrivingLockSWSta/2
  [inp_CanValid_bus] -> slr1_15/1
  slr1_15/1 -> IVIDrivingLockSWSta/3  "<VINP_CANMsgValidIVI1_flg>"
  IVIDrivingLockSWSta/1 -> VINP_IVIDrivingLockSWSta_flg/1  "VINP_IVIDrivingLockSWSta_flg"
  IVIDrivingLockSWSta/2 -> Terminator_15/1
  [BHAL_outputs] -> slr_VHAL_IVIFrTrunkUnlockReqSta_flg/1
  slr_VHAL_IVIFrTrunkUnlockReqSta_flg/1 -> IVIFrTrunkUnlockReqSta/1  "<VHAL_IVIFrTrunkUnlockReqSta_flg>"
  True_VHAL_IVIFrTrunkUnlockReqSta_flg/1 -> IVIFrTrunkUnlockReqSta/2
  [inp_CanValid_bus] -> slr1_16/1
  slr1_16/1 -> IVIFrTrunkUnlockReqSta/3  "<VINP_CANMsgValidIVI1_flg>"
  IVIFrTrunkUnlockReqSta/1 -> VINP_IVIFrTrunkUnlockReqSta_flg/1  "VINP_IVIFrTrunkUnlockReqSta_flg"
  IVIFrTrunkUnlockReqSta/2 -> Terminator_16/1
  [BHAL_outputs] -> slr_VHAL_IVILinkAccReqSta_flg/1
  slr_VHAL_IVILinkAccReqSta_flg/1 -> IVILinkAccReqSta/1  "<VHAL_IVILinkAccReqSta_flg>"
  True_VHAL_IVILinkAccReqSta_flg/1 -> IVILinkAccReqSta/2
  [inp_CanValid_bus] -> slr1_17/1
  slr1_17/1 -> IVILinkAccReqSta/3  "<VINP_CANMsgValidIVI1_flg>"
  IVILinkAccReqSta/1 -> VINP_IVILinkAccReqSta_flg/1  "VINP_IVILinkAccReqSta_flg"
  IVILinkAccReqSta/2 -> Terminator_17/1
  [BHAL_outputs] -> slr_VHAL_IVILinkAccSta_enum/1
  slr_VHAL_IVILinkAccSta_enum/1 -> IVILinkAccSta/1  "<VHAL_IVILinkAccSta_enum>"
  True_VHAL_IVILinkAccSta_enum/1 -> IVILinkAccSta/2
  [inp_CanValid_bus] -> slr1_18/1
  slr1_18/1 -> IVILinkAccSta/3  "<VINP_CANMsgValidIVI1_flg>"
  IVILinkAccSta/1 -> VINP_IVILinkAccSta_enum/1  "VINP_IVILinkAccSta_enum"
  IVILinkAccSta/2 -> Terminator_18/1
  [BHAL_outputs] -> slr_VHAL_IVILinkKeySta_enum/1
  slr_VHAL_IVILinkKeySta_enum/1 -> IVILinkKeySta/1  "<VHAL_IVILinkKeySta_enum>"
  True_VHAL_IVILinkKeySta_enum/1 -> IVILinkKeySta/2
  [inp_CanValid_bus] -> slr1_19/1
  slr1_19/1 -> IVILinkKeySta/3  "<VINP_CANMsgValidIVI1_flg>"
  IVILinkKeySta/1 -> VINP_IVILinkKeySta_enum/1  "VINP_IVILinkKeySta_enum"
  IVILinkKeySta/2 -> Terminator_19/1
  [BHAL_outputs] -> slr_VHAL_IVILocatedSTA_enum/1
  slr_VHAL_IVILocatedSTA_enum/1 -> IVILocatedSTA/1  "<VHAL_IVILocatedSTA_enum>"
  True_VHAL_IVILocatedSTA_enum/1 -> IVILocatedSTA/2
  [inp_CanValid_bus] -> slr1_20/1
  slr1_20/1 -> IVILocatedSTA/3  "<VINP_CANMsgValidIVI1_flg>"
  IVILocatedSTA/1 -> VINP_IVILocatedSTA_enum/1  "VINP_IVILocatedSTA_enum"
  IVILocatedSTA/2 -> Terminator_20/1
  [BHAL_outputs] -> slr_VHAL_IVILockSoundSWSta_flg/1
  slr_VHAL_IVILockSoundSWSta_flg/1 -> IVILockSoundSWSta/1  "<VHAL_IVILockSoundSWSta_flg>"
  True_VHAL_IVILockSoundSWSta_flg/1 -> IVILockSoundSWSta/2
  [inp_CanValid_bus] -> slr1_21/1
  slr1_21/1 -> IVILockSoundSWSta/3  "<VINP_CANMsgValidIVI1_flg>"
  IVILockSoundSWSta/1 -> VINP_IVILockSoundSWSta_flg/1  "VINP_IVILockSoundSWSta_flg"
  IVILockSoundSWSta/2 -> Terminator_21/1
  [BHAL_outputs] -> slr_VHAL_IVISWCVibModeSta_enum/1
  slr_VHAL_IVISWCVibModeSta_enum/1 -> IVISWCVibModeSta/1  "<VHAL_IVISWCVibModeSta_enum>"
  True_VHAL_IVISWCVibModeSta_enum/1 -> IVISWCVibModeSta/2
  [inp_CanValid_bus] -> slr1_22/1
  slr1_22/1 -> IVISWCVibModeSta/3  "<VINP_CANMsgValidIVI1_flg>"
  IVISWCVibModeSta/1 -> VINP_IVISWCVibModeSta_enum/1  "VINP_IVISWCVibModeSta_enum"
  IVISWCVibModeSta/2 -> Terminator_22/1
  [BHAL_outputs] -> slr_VHAL_IVIStoppingUnlockSWSta_flg/1
  slr_VHAL_IVIStoppingUnlockSWSta_flg/1 -> IVIStoppingUnlockSWSta/1  "<VHAL_IVIStoppingUnlockSWSta_flg>"
  True_VHAL_IVIStoppingUnlockSWSta_flg/1 -> IVIStoppingUnlockSWSta/2
  [inp_CanValid_bus] -> slr1_23/1
  slr1_23/1 -> IVIStoppingUnlockSWSta/3  "<VINP_CANMsgValidIVI1_flg>"
  IVIStoppingUnlockSWSta/1 -> VINP_IVIStoppingUnlockSWSta_flg/1  "VINP_IVIStoppingUnlockSWSta_flg"
  IVIStoppingUnlockSWSta/2 -> Terminator_23/1
  [BHAL_outputs] -> slr_VHAL_IVITimeCheck_enum/1
  slr_VHAL_IVITimeCheck_enum/1 -> IVITimeCheck/1  "<VHAL_IVITimeCheck_enum>"
  True_VHAL_IVITimeCheck_enum/1 -> IVITimeCheck/2
  [inp_CanValid_bus] -> slr1_24/1
  slr1_24/1 -> IVITimeCheck/3  "<VINP_CANMsgValidIVI1_flg>"
  IVITimeCheck/1 -> VINP_IVITimeCheck_enum/1  "VINP_IVITimeCheck_enum"
  IVITimeCheck/2 -> Terminator_24/1
  [BHAL_outputs] -> slr_VHAL_IVITimeDay_DAY/1
  slr_VHAL_IVITimeDay_DAY/1 -> IVITimeDay/1  "<VHAL_IVITimeDay_DAY>"
  True_VHAL_IVITimeDay_DAY/1 -> IVITimeDay/2
  [inp_CanValid_bus] -> slr1_25/1
  slr1_25/1 -> IVITimeDay/3  "<VINP_CANMsgValidIVI1_flg>"
  IVITimeDay/1 -> VINP_IVITimeDay_DAY/1  "VINP_IVITimeDay_DAY"
  IVITimeDay/2 -> Terminator_25/1
  [BHAL_outputs] -> slr_VHAL_IVITimeHour_hr/1
  slr_VHAL_IVITimeHour_hr/1 -> IVITimeHour/1  "<VHAL_IVITimeHour_hr>"
  True_VHAL_IVITimeHour_hr/1 -> IVITimeHour/2
  [inp_CanValid_bus] -> slr1_26/1
  slr1_26/1 -> IVITimeHour/3  "<VINP_CANMsgValidIVI1_flg>"
  IVITimeHour/1 -> VINP_IVITimeHour_hr/1  "VINP_IVITimeHour_hr"
  IVITimeHour/2 -> Terminator_26/1
  [BHAL_outputs] -> slr_VHAL_IVITimeMinute_min/1
  slr_VHAL_IVITimeMinute_min/1 -> IVITimeMinute/1  "<VHAL_IVITimeMinute_min>"
  True_VHAL_IVITimeMinute_min/1 -> IVITimeMinute/2
  [inp_CanValid_bus] -> slr1_27/1
  slr1_27/1 -> IVITimeMinute/3  "<VINP_CANMsgValidIVI1_flg>"
  IVITimeMinute/1 -> VINP_IVITimeMinute_min/1  "VINP_IVITimeMinute_min"
  IVITimeMinute/2 -> Terminator_27/1
  [BHAL_outputs] -> slr_VHAL_IVITimeMonth_MONTH/1
  slr_VHAL_IVITimeMonth_MONTH/1 -> IVITimeMonth/1  "<VHAL_IVITimeMonth_MONTH>"
  True_VHAL_IVITimeMonth_MONTH/1 -> IVITimeMonth/2
  [inp_CanValid_bus] -> slr1_28/1
  slr1_28/1 -> IVITimeMonth/3  "<VINP_CANMsgValidIVI1_flg>"
  IVITimeMonth/1 -> VINP_IVITimeMonth_MONTH/1  "VINP_IVITimeMonth_MONTH"
  IVITimeMonth/2 -> Terminator_28/1
  [BHAL_outputs] -> slr_VHAL_IVITimeSecond_s/1
  slr_VHAL_IVITimeSecond_s/1 -> IVITimeSecond/1  "<VHAL_IVITimeSecond_s>"
  True_VHAL_IVITimeSecond_s/1 -> IVITimeSecond/2
  [inp_CanValid_bus] -> slr1_29/1
  slr1_29/1 -> IVITimeSecond/3  "<VINP_CANMsgValidIVI1_flg>"
  IVITimeSecond/1 -> VINP_IVITimeSecond_s/1  "VINP_IVITimeSecond_s"
  IVITimeSecond/2 -> Terminator_29/1
  [BHAL_outputs] -> slr_VHAL_IVITimeYear_YEAR/1
  slr_VHAL_IVITimeYear_YEAR/1 -> IVITimeYear/1  "<VHAL_IVITimeYear_YEAR>"
  True_VHAL_IVITimeYear_YEAR/1 -> IVITimeYear/2
  [inp_CanValid_bus] -> slr1_30/1
  slr1_30/1 -> IVITimeYear/3  "<VINP_CANMsgValidIVI1_flg>"
  IVITimeYear/1 -> VINP_IVITimeYear_YEAR/1  "VINP_IVITimeYear_YEAR"
  IVITimeYear/2 -> Terminator_30/1
  [BHAL_outputs] -> slr_VHAL_IVIWPTCSWSta_flg/1
  slr_VHAL_IVIWPTCSWSta_flg/1 -> IVIWPTCSWSta/1  "<VHAL_IVIWPTCSWSta_flg>"
  True_VHAL_IVIWPTCSWSta_flg/1 -> IVIWPTCSWSta/2
  [inp_CanValid_bus] -> slr1_31/1
  slr1_31/1 -> IVIWPTCSWSta/3  "<VINP_CANMsgValidIVI1_flg>"
  IVIWPTCSWSta/1 -> VINP_IVIWPTCSWSta_flg/1  "VINP_IVIWPTCSWSta_flg"
  IVIWPTCSWSta/2 -> Terminator_31/1
  [BHAL_outputs] -> slr_VHAL_IVIsigScreenReqSta_flg/1
  slr_VHAL_IVIsigScreenReqSta_flg/1 -> IVIsigScreenReqSta/1  "<VHAL_IVIsigScreenReqSta_flg>"
  True_VHAL_IVIsigScreenReqSta_flg/1 -> IVIsigScreenReqSta/2
  [inp_CanValid_bus] -> slr1_32/1
  slr1_32/1 -> IVIsigScreenReqSta/3  "<VINP_CANMsgValidIVI1_flg>"
  IVIsigScreenReqSta/1 -> VINP_IVIsigScreenReqSta_flg/1  "VINP_IVIsigScreenReqSta_flg"
  IVIsigScreenReqSta/2 -> Terminator_32/1
  [BHAL_outputs] -> slr_VHAL_LINKtoDrive_flg/1
  slr_VHAL_LINKtoDrive_flg/1 -> LINKtoDrive/1  "<VHAL_LINKtoDrive_flg>"
  True_VHAL_LINKtoDrive_flg/1 -> LINKtoDrive/2
  [inp_CanValid_bus] -> slr1_33/1
  slr1_33/1 -> LINKtoDrive/3  "<VINP_CANMsgValidIVI1_flg>"
  LINKtoDrive/1 -> VINP_LINKtoDrive_flg/1  "VINP_LINKtoDrive_flg"
  LINKtoDrive/2 -> Terminator_33/1
  [BHAL_outputs] -> slr_VHAL_OpenDrOpenWdoSW_flg/1
  slr_VHAL_OpenDrOpenWdoSW_flg/1 -> OpenDrOpenWdoSW/1  "<VHAL_OpenDrOpenWdoSW_flg>"
  True_VHAL_OpenDrOpenWdoSW_flg/1 -> OpenDrOpenWdoSW/2
  [inp_CanValid_bus] -> slr1_34/1
  slr1_34/1 -> OpenDrOpenWdoSW/3  "<VINP_CANMsgValidIVI1_flg>"
  OpenDrOpenWdoSW/1 -> VINP_OpenDrOpenWdoSW_flg/1  "VINP_OpenDrOpenWdoSW_flg"
  OpenDrOpenWdoSW/2 -> Terminator_34/1
  [BHAL_outputs] -> slr_VHAL_PWCONTINUEUSE_flg/1
  slr_VHAL_PWCONTINUEUSE_flg/1 -> PWCONTINUEUSE/1  "<VHAL_PWCONTINUEUSE_flg>"
  True_VHAL_PWCONTINUEUSE_flg/1 -> PWCONTINUEUSE/2
  [inp_CanValid_bus] -> slr1_35/1
  slr1_35/1 -> PWCONTINUEUSE/3  "<VINP_CANMsgValidIVI1_flg>"
  PWCONTINUEUSE/1 -> VINP_PWCONTINUEUSE_flg/1  "VINP_PWCONTINUEUSE_flg"
  PWCONTINUEUSE/2 -> Terminator_35/1
  [BHAL_outputs] -> slr_VHAL_SmartEcoModeSW_flg/1
  slr_VHAL_SmartEcoModeSW_flg/1 -> SmartEcoModeSW/1  "<VHAL_SmartEcoModeSW_flg>"
  True_VHAL_SmartEcoModeSW_flg/1 -> SmartEcoModeSW/2
  [inp_CanValid_bus] -> slr1_36/1
  slr1_36/1 -> SmartEcoModeSW/3  "<VINP_CANMsgValidIVI1_flg>"
  SmartEcoModeSW/1 -> VINP_SmartEcoModeSW_flg/1  "VINP_SmartEcoModeSW_flg"
  SmartEcoModeSW/2 -> Terminator_36/1
  [BHAL_outputs] -> slr_VHAL_UserSet_enum/1
  slr_VHAL_UserSet_enum/1 -> UserSet/1  "<VHAL_UserSet_enum>"
  True_VHAL_UserSet_enum/1 -> UserSet/2
  [inp_CanValid_bus] -> slr1_37/1
  slr1_37/1 -> UserSet/3  "<VINP_CANMsgValidIVI1_flg>"
  UserSet/1 -> VINP_UserSet_enum/1  "VINP_UserSet_enum"
  UserSet/2 -> Terminator_37/1
